simulink model "SO3_model_AIS"  (R2022a)
settings: Solver=ode4  StartTime=0.0  StopTime=180  FixedStep=0.02  RelTol=1e-3
values from neighbouring files (symbols this model uses):
  alpha = 0.05    [Ini_SO3.m]    (also in Ini_SO3_MixedCZ.m = 0.3; coneNew.m = acos(cosalpha))
  alpha1 = 0.25    [Ini_SO3.m]
  beta = 0.05    [Ini_SO3.m]    (also in Ini_SO3_MixedCZ.m = 0.3)
  deltar = 0.005    [Ini_SO3.m]    (also in Ini_SO3_MixedCZ.m = 0.01; Ini_Usat.m = 0.01)
  G = [1,0,0 ... (first row only)    [Ini_SO3.m]    (also in Ini_SO3_MixedCZ.m; Symmetric test.m = inv(J)*D*E*D')
  J0 = [60 0 -5 ... (first row only)    [Ini_SO3.m]    (also in Ini_SO3_MixedCZ.m)
  J1 = [60 0 -5 ... (first row only)    [Ini_SO3.m]    (also in Ini_SO3_MixedCZ.m)
  J2 = [60 0 -5 ... (first row only)    [Ini_SO3.m]    (also in Ini_SO3_MixedCZ.m)
  J3 = [60 0 -5 ... (first row only)    [Ini_SO3.m]    (also in Ini_SO3_MixedCZ.m)
  K1 = [0.01,0,30,0.2]'    [Ini_SO3.m]    (also in Ini_SO3_MixedCZ.m = [0.01,0,30,0.1]')
  K2 = [0.01,55,55,16,0.001,0.001,0.001]'    [Ini_SO3.m]
  lambda = 0.05    [Ini_SO3.m]    (also in Ini_SO3_MixedCZ.m = 0.3; SO3toThetan.m = diag(lambda))
  lambda1 = 0.25    [Ini_SO3.m]
  N = R/deltar    (= 200)    [Ini_SO3.m]    (also in Ini_SO3_MixedCZ.m; Ini_Usat.m)
  Omega01 = [0.03;0.02;-0.03]    [Ini_SO3.m]    (also in Ini_SO3_MixedCZ.m = [0,0,0])
  Omega02 = [-0.02;0.02;-0.03]    [Ini_SO3.m]    (also in Ini_SO3_MixedCZ.m = [0,0,0])
  Omega03 = [0;0.03;0.04]    [Ini_SO3.m]    (also in Ini_SO3_MixedCZ.m = [0,0,0])
  Omega0d = [0;0;0]    [Ini_SO3.m]    (also in Ini_SO3_MixedCZ.m)
  R = 1    [Ini_SO3.m]    (also in Ini_SO3_MixedCZ.m = 2; Ini_Usat.m = 2; SO3.m = eye(3)+(1-cos(ang))*x2x_hat(x)*x2x_hat(x)+sin(ang)*x2x_hat(x; plot2D.m = tran(lamda_con(j),phi_con(j)))
  R01 = SO3(deg2rad(-80), nd0)    [Ini_SO3.m]    (also in Ini_SO3_MixedCZ.m = SO3(2.387, [0.3145,0.9113,0.2658]'))
  R02 = SO3(deg2rad(40),[0;1;1]/norm([0;1;1]))    [Ini_SO3.m]    (also in Ini_SO3_MixedCZ.m = SO3(1.422, [0.1772,0.9751,-0.1329]'))
  R03 = SO3(deg2rad(-120), nd0)    [Ini_SO3.m]    (also in Ini_SO3_MixedCZ.m = SO3(2.007, [0.2997,0.9415,0.1543]'))
  Rd = SO3(-(2*pi-Angd),nd)    [Ini_SO3.m]    (also in Ini_SO3_MixedCZ.m = SO3(Angd,nd))
  Rd0 = SO3(-(2*pi-Angd0),nd0)    [Ini_SO3.m]    (also in Ini_SO3_MixedCZ.m = SO3(Angd0,nd0))
  thate_T = deg2rad(30)    [Ini_SO3.m]    (also in Ini_SO3_MixedCZ.m = deg2rad(10))
  X = zeros(4,4)    [Ini_SO3.m]    (also in Ini_SO3_MixedCZ.m; coneNew.m = R .* cos(A))
undefined symbols (not defined in the file or in its folder): deg, rad, s
libraries: matrix_library x7, aerolibconvert2 x5
(part 1 of 2)
settings Model: Creator=Zeyu  LastModifiedBy=泽禹
settings DebuggingCC: UnconnectedInputMsg=warning  UnconnectedOutputMsg=warning  UnconnectedLineMsg=warning  UnderSpecifiedDimensionMsg=warning
settings RTWCC: DLArmComputeVersion=19.05

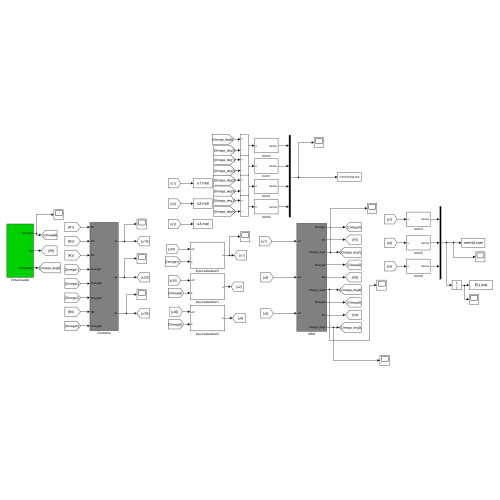
[thumbnail: Simulink's stored preview of the top-level diagram]
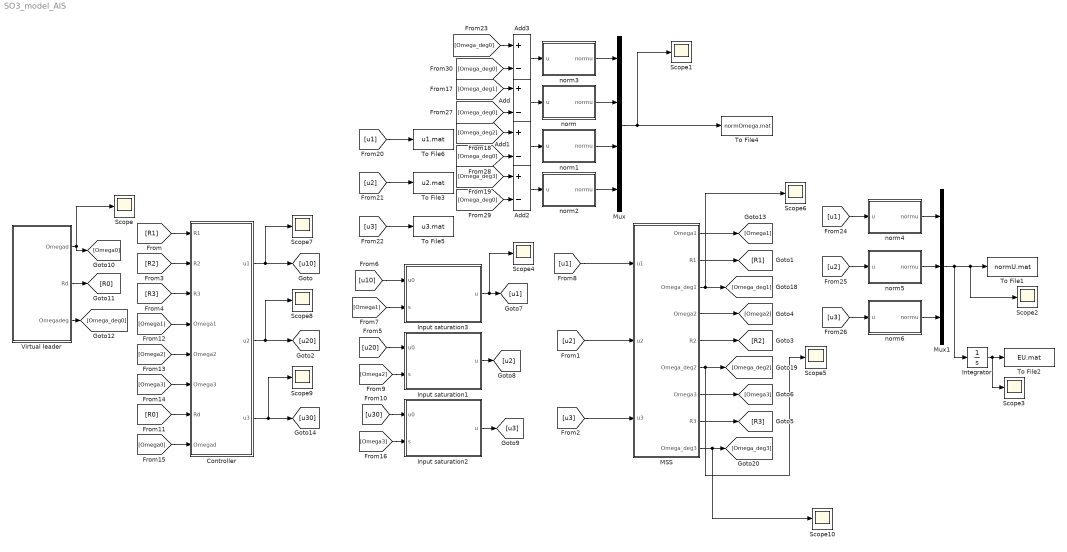
== system SO3_model_AIS ==
  Add{,1..3} (4 alike) : Sum  Inputs=+-
  Controller : Subsystem
  Input saturation1 : Subsystem
  Input saturation2 : Subsystem
  Input saturation3 : Subsystem
  Integrator : Integrator
  MSS : Subsystem
  Mux : Mux
  Mux1 : Mux  Inputs=3
  Scope{,1..10} (11 alike) : Scope
  To File1 : ToFile  Filename=normU.mat  MatrixName=normU
  To File2 : ToFile  Filename=EU.mat  MatrixName=EU
  To File3 : ToFile  Filename=u2.mat  MatrixName=u2
  To File4 : ToFile  Filename=normOmega.mat  MatrixName=normOmega
  To File5 : ToFile  Filename=u3.mat  MatrixName=u3
  To File6 : ToFile  Filename=u1.mat  MatrixName=u1
  Virtual leader : Subsystem
  norm : Subsystem
  norm1 : Subsystem
  norm2 : Subsystem
  norm3 : Subsystem
  norm4 : Subsystem
  norm5 : Subsystem
  norm6 : Subsystem
  wires:
  Virtual leader/1(Omegad) -> [Omega0], Scope/1
  Virtual leader/2(Rd) -> [R0]
  [R1] -> Controller/1(R1)
  [R2] -> Controller/2(R2)
  [R3] -> Controller/3(R3)
  [Omega1] -> Controller/4(Omega1)
  [Omega2] -> Controller/5(Omega2)
  [Omega3] -> Controller/6(Omega3)
  [R0] -> Controller/7(Rd)
  [Omega0] -> Controller/8(Omegad)
  Controller/1(u1) -> Scope7/1, [u10]
  Controller/2(u2) -> Scope8/1, [u20]
  Controller/3(u3) -> Scope9/1, [u30]
  MSS/1(Omega1) -> [Omega1]
  MSS/2(R1) -> [R1]
  MSS/3(Omega_deg1) -> Scope6/1, [Omega_deg1]
  MSS/4(Omega2) -> [Omega2]
  MSS/5(R2) -> [R2]
  MSS/7(Omega3) -> [Omega3]
  MSS/8(R3) -> [R3]
  MSS/9(Omega_deg3) -> Scope10/1, [Omega_deg3]
  [u10] -> Input saturation3/1(u0)
  [Omega1] -> Input saturation3/2(s)
  Input saturation3/1(u) -> Scope4/1, [u1]
  [u20] -> Input saturation1/1(u0)
  [Omega2] -> Input saturation1/2(s)
  Input saturation1/1(u) -> [u2]
  [u30] -> Input saturation2/1(u0)
  [Omega3] -> Input saturation2/2(s)
  Input saturation2/1(u) -> [u3]
  [u1] -> MSS/1(u1)
  [u2] -> MSS/2(u2)
  [u3] -> MSS/3(u3)
  MSS/6(Omega_deg2) -> Scope5/1, [Omega_deg2]
  [u1] -> To File6/1
  [u3] -> To File5/1
  [u2] -> To File3/1
  Virtual leader/3(Omegadeg) -> [Omega_deg0]
  norm3/1(normu) -> Mux/1
  norm/1(normu) -> Mux/2
  norm1/1(normu) -> Mux/3
  norm2/1(normu) -> Mux/4
  Mux/1 -> Scope1/1, To File4/1
  norm4/1(normu) -> Mux1/1
  norm5/1(normu) -> Mux1/2
  norm6/1(normu) -> Mux1/3
  [u1] -> norm4/1(u)
  [u2] -> norm5/1(u)
  [u3] -> norm6/1(u)
  Mux1/1 -> Integrator/1, Scope2/1, To File1/1
  Integrator/1 -> Scope3/1, To File2/1
  [Omega_deg1] -> Add/1
  Add/1 -> norm/1(u)
  [Omega_deg0] -> Add/2
  [Omega_deg0] -> Add1/2
  [Omega_deg2] -> Add1/1
  Add1/1 -> norm1/1(u)
  [Omega_deg0] -> Add2/2
  [Omega_deg3] -> Add2/1
  Add2/1 -> norm2/1(u)
  [Omega_deg0] -> Add3/2
  Add3/1 -> norm3/1(u)
  [Omega_deg0] -> Add3/1

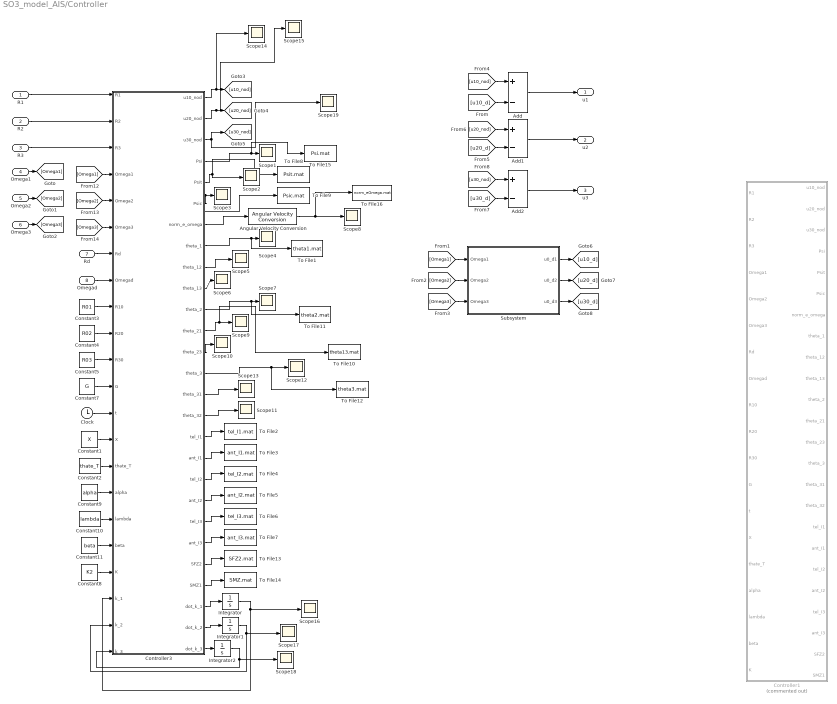
== system SO3_model_AIS/Controller ==
  R1 : Inport
  R2 : Inport  Port=2
  R3 : Inport  Port=3
  Omega1 : Inport  Port=4
  Omega2 : Inport  Port=5
  Omega3 : Inport  Port=6
  Rd : Inport  Port=7
  Omegad : Inport  Port=8
  Add : Sum  Inputs=+-
  Add1 : Sum  Inputs=+-
  Add2 : Sum  Inputs=+-
  Angular Velocity Conversion : aerolibconvert2/Angular Velocity Conversion  IU=rad/s  OU=deg/s
  Clock : Clock
  Constant1 : Constant  Value=X
  Constant10 : Constant  Value=lambda
  Constant11 : Constant  Value=beta
  Constant2 : Constant  Value=thate_T
  Constant3 : Constant  Value=R01
  Constant4 : Constant  Value=R02
  Constant5 : Constant  Value=R03
  Constant7 : Constant  Value=G
  Constant8 : Constant  Value=K2
  Constant9 : Constant  Value=alpha
  Controller1 : MATLAB Function  Commented=on  TreatAsAtomicUnit=on
  Controller3 : MATLAB Function  TreatAsAtomicUnit=on
  Integrator : Integrator  InitialCondition=[0.05;0.05;0.05]
  Integrator1 : Integrator  InitialCondition=[0.05;0.05;0.05]
  Integrator2 : Integrator  InitialCondition=[0.05;0.05;0.05]
  Scope{1..19} (19 alike) : Scope
  Subsystem : Subsystem
  To File1 : ToFile  Filename=theta1.mat  MatrixName=theta1
  To File10 : ToFile  Filename=theta13.mat  MatrixName=theta13
  To File11 : ToFile  Filename=theta2.mat  MatrixName=theta2
  To File12 : ToFile  Filename=theta3.mat  MatrixName=theta3
  To File13 : ToFile  Filename=SFZ2.mat  MatrixName=SFZ2
  To File14 : ToFile  Filename=SMZ.mat  MatrixName=SMZ
  To File15 : ToFile  Filename=Psi.mat  MatrixName=Psi
  To File16 : ToFile  Filename=norm_eOmega.mat  MatrixName=norm_eOmega
  To File2 : ToFile  Filename=tel_I1.mat  MatrixName=tel_I1
  To File3 : ToFile  Filename=ant_I1.mat  MatrixName=ant_I1
  To File4 : ToFile  Filename=tel_I2.mat  MatrixName=tel_I2
  To File5 : ToFile  Filename=ant_I2.mat  MatrixName=ant_I2
  To File6 : ToFile  Filename=tel_I3.mat  MatrixName=tel_I3
  To File7 : ToFile  Filename=ant_I3.mat  MatrixName=ant_I3
  To File8 : ToFile  Filename=Psit.mat  MatrixName=Psit
  To File9 : ToFile  Filename=Psic.mat  MatrixName=Psic
  u1 : Outport
  u2 : Outport  Port=2
  u3 : Outport  Port=3
  wires:
  Constant7/1 -> Controller3/12(G)
  Clock/1 -> Controller3/13(t)
  Constant8/1 -> Controller3/19(K)
  Constant4/1 -> Controller3/10(R20)
  Constant10/1 -> Controller3/17(lambda)
  Constant3/1 -> Controller3/9(R10)
  Omegad/1 -> Controller3/8(Omegad)
  R2/1 -> Controller3/2(R2)
  Constant11/1 -> Controller3/18(beta)
  Constant2/1 -> Controller3/15(thate_T)
  Constant1/1 -> Controller3/14(X)
  Controller3/7(norm_e_omega) -> Angular Velocity Conversion/1
  Constant9/1 -> Controller3/16(alpha)
  Rd/1 -> Controller3/7(Rd)
  Controller3/4(Psi) -> Scope1/1, To File15/1
  Controller3/6(Psic) -> To File9/1, Scope3/1
  R3/1 -> Controller3/3(R3)
  Constant5/1 -> Controller3/11(R30)
  R1/1 -> Controller3/1(R1)
  [Omega2] -> Controller3/5(Omega2)
  [Omega1] -> Controller3/4(Omega1)
  [Omega3] -> Controller3/6(Omega3)
  Omega1/1 -> [Omega1]
  Omega2/1 -> [Omega2]
  Omega3/1 -> [Omega3]
  [Omega1] -> Subsystem/1(Omega1)
  [Omega2] -> Subsystem/2(Omega2)
  [Omega3] -> Subsystem/3(Omega3)
  Add/1 -> u1/1
  Add1/1 -> u2/1
  Add2/1 -> u3/1
  Controller3/1(u10_nod) -> Scope14/1, [u10_nod]
  Controller3/2(u20_nod) -> Scope15/1, [u20_nod]
  Controller3/3(u30_nod) -> [u30_nod], Scope19/1
  Subsystem/2(u0_d2) -> [u20_d]
  Subsystem/1(u0_d1) -> [u10_d]
  Subsystem/3(u0_d3) -> [u30_d]
  [u10_d] -> Add/2
  [u10_nod] -> Add/1
  [u20_d] -> Add1/2
  [u20_nod] -> Add1/1
  [u30_d] -> Add2/2
  [u30_nod] -> Add2/1
  Controller3/17(tel_I1) -> To File2/1
  Controller3/18(ant_I1) -> To File3/1
  Controller3/19(tel_I2) -> To File4/1
  Controller3/20(ant_I2) -> To File5/1
  Controller3/21(tel_I3) -> To File6/1
  Controller3/22(ant_I3) -> To File7/1
  Controller3/8(theta_1) -> To File1/1, Scope4/1
  Controller3/9(theta_12) -> Scope5/1
  Controller3/12(theta_21) -> To File10/1, Scope9/1
  Controller3/13(theta_23) -> Scope10/1
  Controller3/16(theta_32) -> Scope11/1
  Controller3/15(theta_31) -> Scope13/1
  Controller3/14(theta_3) -> To File12/1, Scope12/1
  Controller3/5(Psit) -> Scope2/1, To File8/1
  Controller3/10(theta_13) -> Scope6/1
  Controller3/11(theta_2) -> To File11/1, Scope7/1
  Controller3/23(SFZ2) -> To File13/1
  Controller3/24(SMZ1) -> To File14/1
  Controller3/25(dot_k_1) -> Integrator/1
  Integrator/1 -> Scope16/1, Controller3/20(k_1)
  Controller3/26(dot_k_2) -> Integrator1/1
  Integrator1/1 -> Scope17/1, Controller3/21(k_2)
  Controller3/27(dot_k_3) -> Integrator2/1
  Integrator2/1 -> Scope18/1, Controller3/22(k_3)
  Angular Velocity Conversion/1 -> To File16/1, Scope8/1

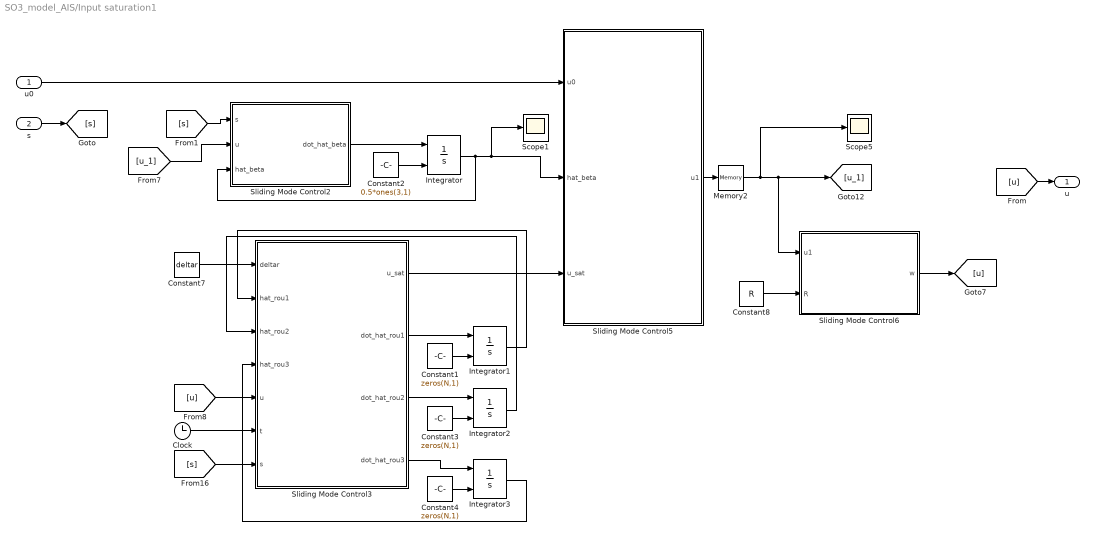
== system SO3_model_AIS/Input saturation1 ==
  u0 : Inport
  s : Inport  Port=2
  Clock : Clock
  Constant1 : Constant  Value=zeros(N,1)
  Constant2 : Constant  Value=0.5*ones(3,1)
  Constant3 : Constant  Value=zeros(N,1)
  Constant4 : Constant  Value=zeros(N,1)
  Constant7 : Constant  Value=deltar
  Constant8 : Constant  Value=R
  Integrator{,1..3} (4 alike) : Integrator  InitialConditionSource=external
  Memory2 : Memory
  Scope1 : Scope
  Scope5 : Scope
  Sliding Mode Control2 : MATLAB Function  TreatAsAtomicUnit=on
  Sliding Mode Control3 : MATLAB Function  TreatAsAtomicUnit=on
  Sliding Mode Control5 : MATLAB Function  TreatAsAtomicUnit=on
  Sliding Mode Control6 : MATLAB Function  TreatAsAtomicUnit=on
  u : Outport
  wires:
  [s] -> Sliding Mode Control2/1(s)
  s/1 -> [s]
  [u] -> u/1
  u0/1 -> Sliding Mode Control5/1(u0)
  Constant8/1 -> Sliding Mode Control6/2(R)
  Memory2/1 -> Scope5/1, Sliding Mode Control6/1(u1), [u_1]
  Sliding Mode Control6/1(w) -> [u]
  [u_1] -> Sliding Mode Control2/2(u)
  Sliding Mode Control5/1(u1) -> Memory2/1
  Sliding Mode Control2/1(dot_hat_beta) -> Integrator/1
  Constant2/1 -> Integrator/2
  Integrator/1 -> Sliding Mode Control2/3(hat_beta), Scope1/1, Sliding Mode Control5/2(hat_beta)
  [u] -> Sliding Mode Control3/5(u)
  Integrator1/1 -> Sliding Mode Control3/2(hat_rou1)
  Sliding Mode Control3/3(dot_hat_rou2) -> Integrator2/1
  [s] -> Sliding Mode Control3/7(s)
  Constant7/1 -> Sliding Mode Control3/1(deltar)
  Constant4/1 -> Integrator3/2
  Integrator2/1 -> Sliding Mode Control3/3(hat_rou2)
  Sliding Mode Control3/4(dot_hat_rou3) -> Integrator3/1
  Integrator3/1 -> Sliding Mode Control3/4(hat_rou3)
  Sliding Mode Control3/2(dot_hat_rou1) -> Integrator1/1
  Clock/1 -> Sliding Mode Control3/6(t)
  Constant1/1 -> Integrator1/2
  Sliding Mode Control3/1(u_sat) -> Sliding Mode Control5/3(u_sat)
  Constant3/1 -> Integrator2/2

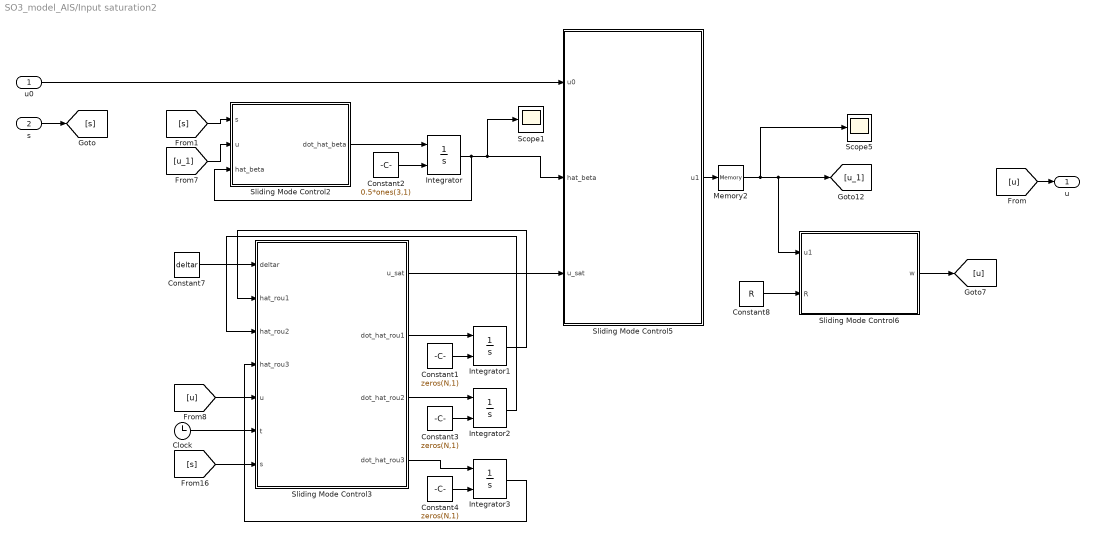
== system SO3_model_AIS/Input saturation2 ==
  u0 : Inport
  s : Inport  Port=2
  Clock : Clock
  Constant1 : Constant  Value=zeros(N,1)
  Constant2 : Constant  Value=0.5*ones(3,1)
  Constant3 : Constant  Value=zeros(N,1)
  Constant4 : Constant  Value=zeros(N,1)
  Constant7 : Constant  Value=deltar
  Constant8 : Constant  Value=R
  Integrator{,1..3} (4 alike) : Integrator  InitialConditionSource=external
  Memory2 : Memory
  Scope1 : Scope
  Scope5 : Scope
  Sliding Mode Control2 : MATLAB Function  TreatAsAtomicUnit=on
  Sliding Mode Control3 : MATLAB Function  TreatAsAtomicUnit=on
  Sliding Mode Control5 : MATLAB Function  TreatAsAtomicUnit=on
  Sliding Mode Control6 : MATLAB Function  TreatAsAtomicUnit=on
  u : Outport
  wires:
  Constant2/1 -> Integrator/2
  Sliding Mode Control2/1(dot_hat_beta) -> Integrator/1
  Sliding Mode Control5/1(u1) -> Memory2/1
  [u_1] -> Sliding Mode Control2/2(u)
  Sliding Mode Control6/1(w) -> [u]
  Memory2/1 -> Sliding Mode Control6/1(u1), [u_1], Scope5/1
  Constant8/1 -> Sliding Mode Control6/2(R)
  [u] -> u/1
  s/1 -> [s]
  [s] -> Sliding Mode Control2/1(s)
  Integrator/1 -> Sliding Mode Control2/3(hat_beta), Scope1/1, Sliding Mode Control5/2(hat_beta)
  u0/1 -> Sliding Mode Control5/1(u0)
  [u] -> Sliding Mode Control3/5(u)
  Integrator1/1 -> Sliding Mode Control3/2(hat_rou1)
  Sliding Mode Control3/3(dot_hat_rou2) -> Integrator2/1
  [s] -> Sliding Mode Control3/7(s)
  Constant7/1 -> Sliding Mode Control3/1(deltar)
  Constant4/1 -> Integrator3/2
  Integrator2/1 -> Sliding Mode Control3/3(hat_rou2)
  Sliding Mode Control3/4(dot_hat_rou3) -> Integrator3/1
  Sliding Mode Control3/2(dot_hat_rou1) -> Integrator1/1
  Clock/1 -> Sliding Mode Control3/6(t)
  Constant1/1 -> Integrator1/2
  Sliding Mode Control3/1(u_sat) -> Sliding Mode Control5/3(u_sat)
  Constant3/1 -> Integrator2/2
  Integrator3/1 -> Sliding Mode Control3/4(hat_rou3)

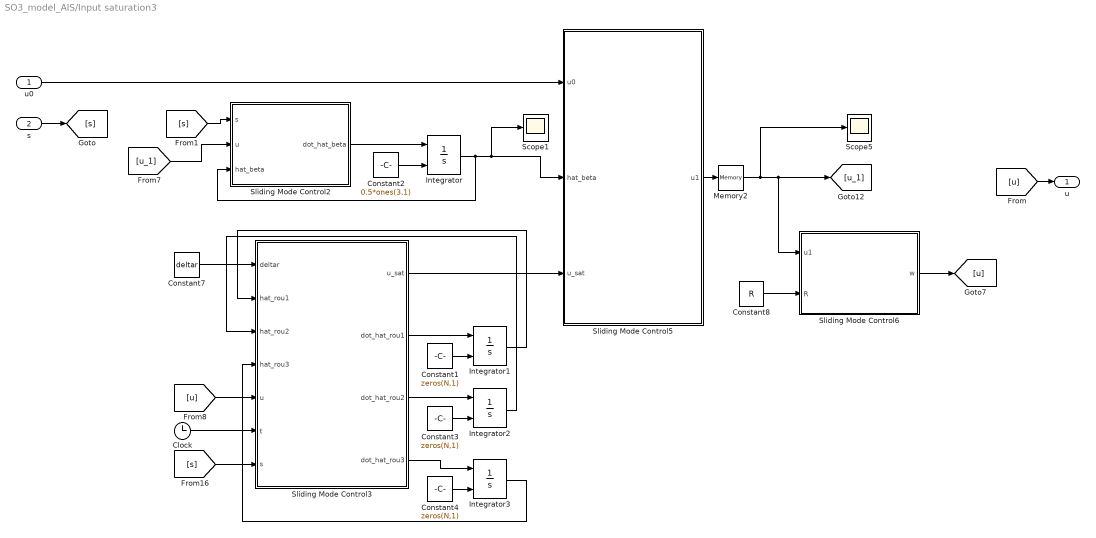
== system SO3_model_AIS/Input saturation3 ==
  u0 : Inport
  s : Inport  Port=2
  Clock : Clock
  Constant1 : Constant  Value=zeros(N,1)
  Constant2 : Constant  Value=0.5*ones(3,1)
  Constant3 : Constant  Value=zeros(N,1)
  Constant4 : Constant  Value=zeros(N,1)
  Constant7 : Constant  Value=deltar
  Constant8 : Constant  Value=R
  Integrator{,1..3} (4 alike) : Integrator  InitialConditionSource=external
  Memory2 : Memory
  Scope1 : Scope
  Scope5 : Scope
  Sliding Mode Control2 : MATLAB Function  TreatAsAtomicUnit=on
  Sliding Mode Control3 : MATLAB Function  TreatAsAtomicUnit=on
  Sliding Mode Control5 : MATLAB Function  TreatAsAtomicUnit=on
  Sliding Mode Control6 : MATLAB Function  TreatAsAtomicUnit=on
  u : Outport
  wires:
  Constant3/1 -> Integrator2/2
  Sliding Mode Control3/1(u_sat) -> Sliding Mode Control5/3(u_sat)
  Constant1/1 -> Integrator1/2
  Clock/1 -> Sliding Mode Control3/6(t)
  Sliding Mode Control3/2(dot_hat_rou1) -> Integrator1/1
  Integrator3/1 -> Sliding Mode Control3/4(hat_rou3)
  Sliding Mode Control3/4(dot_hat_rou3) -> Integrator3/1
  Integrator2/1 -> Sliding Mode Control3/3(hat_rou2)
  Constant4/1 -> Integrator3/2
  Constant7/1 -> Sliding Mode Control3/1(deltar)
  [s] -> Sliding Mode Control3/7(s)
  Sliding Mode Control3/3(dot_hat_rou2) -> Integrator2/1
  Integrator1/1 -> Sliding Mode Control3/2(hat_rou1)
  [u] -> Sliding Mode Control3/5(u)
  Integrator/1 -> Sliding Mode Control5/2(hat_beta), Scope1/1, Sliding Mode Control2/3(hat_beta)
  Constant2/1 -> Integrator/2
  Sliding Mode Control2/1(dot_hat_beta) -> Integrator/1
  Sliding Mode Control5/1(u1) -> Memory2/1
  [u_1] -> Sliding Mode Control2/2(u)
  Sliding Mode Control6/1(w) -> [u]
  Memory2/1 -> [u_1], Sliding Mode Control6/1(u1), Scope5/1
  Constant8/1 -> Sliding Mode Control6/2(R)
  u0/1 -> Sliding Mode Control5/1(u0)
  [u] -> u/1
  s/1 -> [s]
  [s] -> Sliding Mode Control2/1(s)

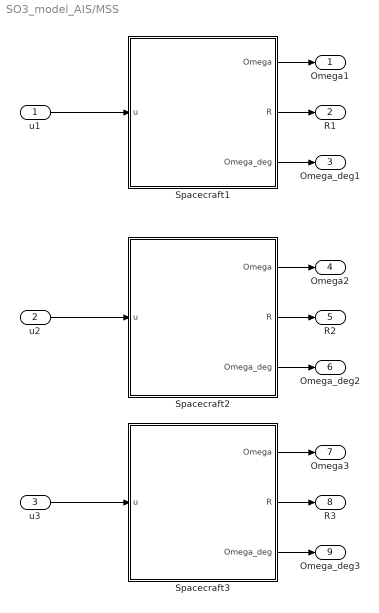
== system SO3_model_AIS/MSS ==
  u1 : Inport
  u2 : Inport  Port=2
  u3 : Inport  Port=3
  Spacecraft1 : Subsystem
  Spacecraft2 : Subsystem
  Spacecraft3 : Subsystem
  Omega1 : Outport
  R1 : Outport  Port=2
  Omega_deg1 : Outport  Port=3
  Omega2 : Outport  Port=4
  R2 : Outport  Port=5
  Omega_deg2 : Outport  Port=6
  Omega3 : Outport  Port=7
  R3 : Outport  Port=8
  Omega_deg3 : Outport  Port=9
  wires:
  Spacecraft3/2(R) -> R3/1
  Spacecraft1/1(Omega) -> Omega1/1
  u1/1 -> Spacecraft1/1(u)
  Spacecraft2/3(Omega_deg) -> Omega_deg2/1
  Spacecraft2/1(Omega) -> Omega2/1
  u3/1 -> Spacecraft3/1(u)
  Spacecraft1/2(R) -> R1/1
  Spacecraft3/3(Omega_deg) -> Omega_deg3/1
  Spacecraft3/1(Omega) -> Omega3/1
  Spacecraft1/3(Omega_deg) -> Omega_deg1/1
  u2/1 -> Spacecraft2/1(u)
  Spacecraft2/2(R) -> R2/1

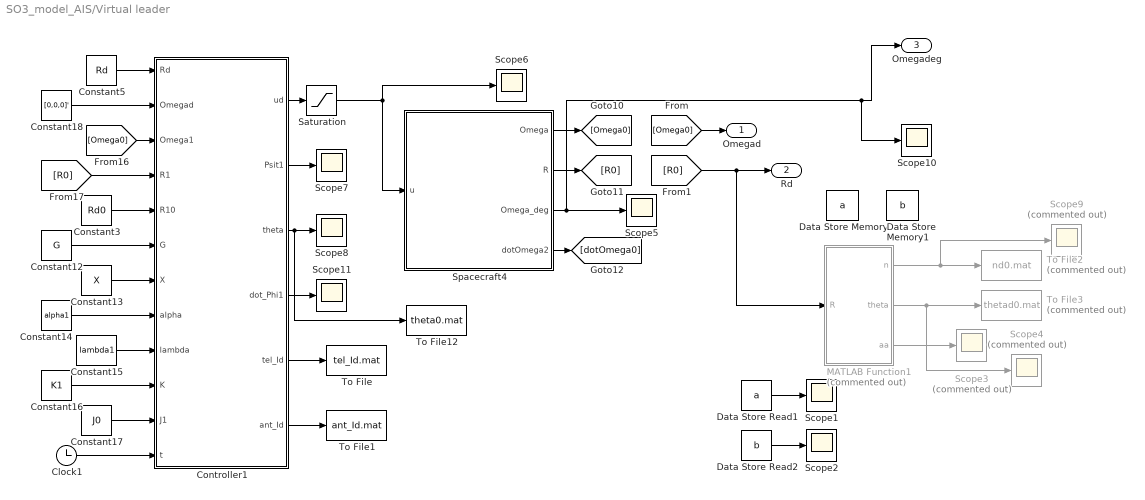
== system SO3_model_AIS/Virtual leader ==
  Clock1 : Clock
  Constant12 : Constant  Value=G
  Constant13 : Constant  Value=X
  Constant14 : Constant  Value=alpha1
  Constant15 : Constant  Value=lambda1
  Constant16 : Constant  Value=K1
  Constant17 : Constant  Value=J0
  Constant18 : Constant  Value=[0,0,0]'
  Constant3 : Constant  Value=Rd0
  Constant5 : Constant  Value=Rd
  Controller1 : MATLAB Function  TreatAsAtomicUnit=on
  Data Store Memory : DataStoreMemory  DataStoreName=a  ReadBeforeWriteMsg=warning  WriteAfterWriteMsg=warning  WriteAfterReadMsg=warning  InitialValue=ones(4,1)  ShowAdditionalParam=off  OutDataTypeStr=double
  Data Store Memory1 : DataStoreMemory  DataStoreName=b  ReadBeforeWriteMsg=warning  WriteAfterWriteMsg=warning  WriteAfterReadMsg=warning  InitialValue=zeros(4,1)  ShowAdditionalParam=off  OutDataTypeStr=double
  Data Store Read1 : DataStoreRead  DataStoreName=a  IndexOptions=Index vector (dialog)  Indices=1  OutputSizes=1
  Data Store Read2 : DataStoreRead  DataStoreName=b  IndexOptions=Index vector (dialog)  Indices=1  OutputSizes=1
  MATLAB Function1 : MATLAB Function  Commented=on  TreatAsAtomicUnit=on
  Saturation : Saturate  UpperLimit=1  LowerLimit=-1
  Scope{1..2,5..8,10..11} (8 alike) : Scope
  Scope3 : Scope  Commented=on
  Scope4 : Scope  Commented=on
  Scope9 : Scope  Commented=on
  Spacecraft4 : Subsystem
  To File : ToFile  Filename=tel_Id.mat  MatrixName=tel_Id
  To File1 : ToFile  Filename=ant_Id.mat  MatrixName=ant_Id
  To File12 : ToFile  Filename=theta0.mat  MatrixName=theta0
  To File2 : ToFile  Commented=on  Filename=nd0.mat  MatrixName=nd0
  To File3 : ToFile  Commented=on  Filename=thetad0.mat  MatrixName=thetad0
  Omegad : Outport
  Rd : Outport  Port=2
  Omegadeg : Outport  Port=3
  wires:
  Spacecraft4/4(dotOmega2) -> [dotOmega0]
  [R0] -> Controller1/4(R1)
  Controller1/1(ud) -> Saturation/1
  Constant16/1 -> Controller1/10(K)
  Constant12/1 -> Controller1/6(G)
  Constant18/1 -> Controller1/2(Omegad)
  Constant17/1 -> Controller1/11(J1)
  Constant5/1 -> Controller1/1(Rd)
  Constant14/1 -> Controller1/8(alpha)
  Constant15/1 -> Controller1/9(lambda)
  Constant13/1 -> Controller1/7(X)
  Clock1/1 -> Controller1/12(t)
  [Omega0] -> Controller1/3(Omega1)
  Controller1/4(dot_Phi1) -> Scope11/1
  Controller1/2(Psit1) -> Scope7/1
  Spacecraft4/2(R) -> [R0]
  Spacecraft4/1(Omega) -> [Omega0]
  [Omega0] -> Omegad/1
  Constant3/1 -> Controller1/5(R10)
  Data Store Read1/1 -> Scope1/1
  Data Store Read2/1 -> Scope2/1
  Saturation/1 -> Spacecraft4/1(u), Scope6/1
  Controller1/5(tel_Id) -> To File/1
  Controller1/6(ant_Id) -> To File1/1
  [R0] -> MATLAB Function1/1(R), Rd/1
  MATLAB Function1/1(n) -> Scope9/1, To File2/1
  MATLAB Function1/2(theta) -> Scope4/1, To File3/1
  MATLAB Function1/3(aa) -> Scope3/1
  Controller1/3(theta) -> To File12/1, Scope8/1
  Spacecraft4/3(Omega_deg) -> Scope5/1, Scope10/1, Omegadeg/1

== system SO3_model_AIS/norm ==
  u : Inport
  Matrix Square : matrix_library/Matrix Square  OutMin=[]  OutMax=[]
      settings: SourceProductBaseCode=DS
  Sqrt : Sqrt
  normu : Outport
  wires:
  Sqrt/1 -> normu/1
  Matrix Square/1 -> Sqrt/1
  u/1 -> Matrix Square/1

== system SO3_model_AIS/norm1 ==
  u : Inport
  Matrix Square : matrix_library/Matrix Square  OutMin=[]  OutMax=[]
      settings: SourceProductBaseCode=DS
  Sqrt : Sqrt
  normu : Outport
  wires:
  Sqrt/1 -> normu/1
  Matrix Square/1 -> Sqrt/1
  u/1 -> Matrix Square/1

== system SO3_model_AIS/norm2 ==
  u : Inport
  Matrix Square : matrix_library/Matrix Square  OutMin=[]  OutMax=[]
      settings: SourceProductBaseCode=DS
  Sqrt : Sqrt
  normu : Outport
  wires:
  Sqrt/1 -> normu/1
  Matrix Square/1 -> Sqrt/1
  u/1 -> Matrix Square/1

== system SO3_model_AIS/norm3 ==
  u : Inport
  Matrix Square : matrix_library/Matrix Square  OutMin=[]  OutMax=[]
      settings: SourceProductBaseCode=DS
  Sqrt : Sqrt
  normu : Outport
  wires:
  u/1 -> Matrix Square/1
  Matrix Square/1 -> Sqrt/1
  Sqrt/1 -> normu/1

== system SO3_model_AIS/norm4 ==
  u : Inport
  Matrix Square : matrix_library/Matrix Square  OutMin=[]  OutMax=[]
      settings: SourceProductBaseCode=DS
  Sqrt : Sqrt
  normu : Outport
  wires:
  Sqrt/1 -> normu/1
  Matrix Square/1 -> Sqrt/1
  u/1 -> Matrix Square/1

== system SO3_model_AIS/norm5 ==
  u : Inport
  Matrix Square : matrix_library/Matrix Square  OutMin=[]  OutMax=[]
      settings: SourceProductBaseCode=DS
  Sqrt : Sqrt
  normu : Outport
  wires:
  u/1 -> Matrix Square/1
  Matrix Square/1 -> Sqrt/1
  Sqrt/1 -> normu/1

== system SO3_model_AIS/norm6 ==
  u : Inport
  Matrix Square : matrix_library/Matrix Square  OutMin=[]  OutMax=[]
      settings: SourceProductBaseCode=DS
  Sqrt : Sqrt
  normu : Outport
  wires:
  Sqrt/1 -> normu/1
  Matrix Square/1 -> Sqrt/1
  u/1 -> Matrix Square/1

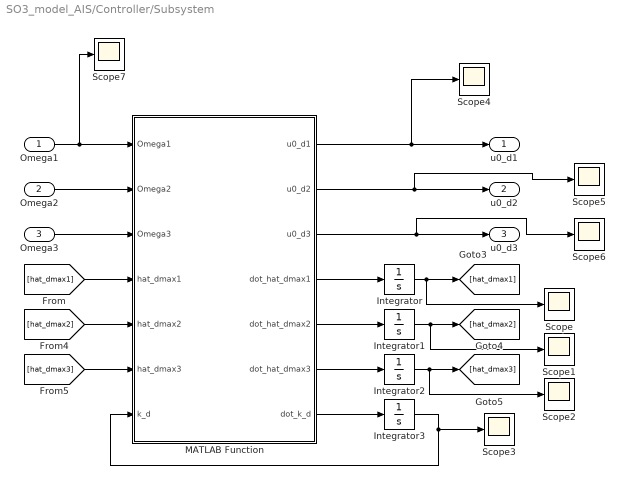
== system SO3_model_AIS/Controller/Subsystem ==
  Omega1 : Inport
  Omega2 : Inport  Port=2
  Omega3 : Inport  Port=3
  Integrator : Integrator
  Integrator1 : Integrator
  Integrator2 : Integrator
  Integrator3 : Integrator  InitialCondition=0.05*ones(3,1)
  MATLAB Function : MATLAB Function  TreatAsAtomicUnit=on
  Scope{,1..7} (8 alike) : Scope
  u0_d1 : Outport
  u0_d2 : Outport  Port=2
  u0_d3 : Outport  Port=3
  wires:
  Integrator2/1 -> [hat_dmax3], Scope2/1
  Integrator1/1 -> Scope1/1, [hat_dmax2]
  MATLAB Function/1(u0_d1) -> Scope4/1, u0_d1/1
  MATLAB Function/4(dot_hat_dmax1) -> Integrator/1
  [hat_dmax2] -> MATLAB Function/5(hat_dmax2)
  MATLAB Function/5(dot_hat_dmax2) -> Integrator1/1
  Omega2/1 -> MATLAB Function/2(Omega2)
  Omega1/1 -> Scope7/1, MATLAB Function/1(Omega1)
  [hat_dmax3] -> MATLAB Function/6(hat_dmax3)
  MATLAB Function/6(dot_hat_dmax3) -> Integrator2/1
  Integrator/1 -> Scope/1, [hat_dmax1]
  [hat_dmax1] -> MATLAB Function/4(hat_dmax1)
  MATLAB Function/2(u0_d2) -> Scope5/1, u0_d2/1
  MATLAB Function/3(u0_d3) -> Scope6/1, u0_d3/1
  Omega3/1 -> MATLAB Function/3(Omega3)
  MATLAB Function/7(dot_k_d) -> Integrator3/1
  Integrator3/1 -> MATLAB Function/7(k_d), Scope3/1

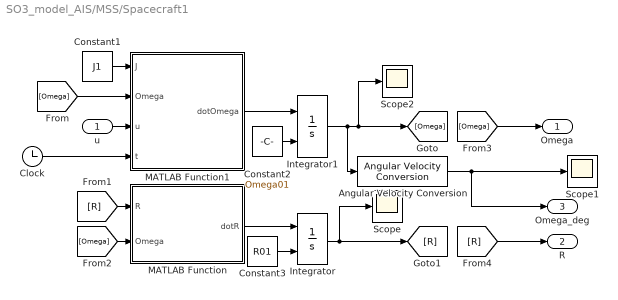
== system SO3_model_AIS/MSS/Spacecraft1 ==
  u : Inport
  Angular Velocity Conversion : aerolibconvert2/Angular Velocity Conversion  IU=rad/s  OU=deg/s
  Clock : Clock
  Constant1 : Constant  Value=J1
  Constant2 : Constant  Value=Omega01
  Constant3 : Constant  Value=R01
  Integrator : Integrator  InitialConditionSource=external
  Integrator1 : Integrator  InitialConditionSource=external
  MATLAB Function : MATLAB Function  TreatAsAtomicUnit=on
  MATLAB Function1 : MATLAB Function  TreatAsAtomicUnit=on
  Scope : Scope
  Scope1 : Scope
  Scope2 : Scope
  Omega : Outport
  R : Outport  Port=2
  Omega_deg : Outport  Port=3
  wires:
  Constant3/1 -> Integrator/2
  Integrator/1 -> [R], Scope/1
  Constant1/1 -> MATLAB Function1/1(J)
  Integrator1/1 -> Scope2/1, [Omega], Angular Velocity Conversion/1
  MATLAB Function1/1(dotOmega) -> Integrator1/1
  [Omega] -> MATLAB Function/2(Omega)
  MATLAB Function/1(dotR) -> Integrator/1
  Constant2/1 -> Integrator1/2
  [Omega] -> MATLAB Function1/2(Omega)
  [R] -> MATLAB Function/1(R)
  Angular Velocity Conversion/1 -> Omega_deg/1, Scope1/1
  u/1 -> MATLAB Function1/3(u)
  [Omega] -> Omega/1
  [R] -> R/1
  Clock/1 -> MATLAB Function1/4(t)

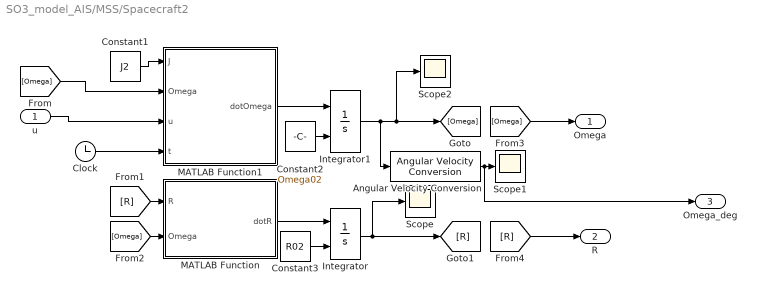
== system SO3_model_AIS/MSS/Spacecraft2 ==
  u : Inport
  Angular Velocity Conversion : aerolibconvert2/Angular Velocity Conversion  IU=rad/s  OU=deg/s
  Clock : Clock
  Constant1 : Constant  Value=J2
  Constant2 : Constant  Value=Omega02
  Constant3 : Constant  Value=R02
  Integrator : Integrator  InitialConditionSource=external
  Integrator1 : Integrator  InitialConditionSource=external
  MATLAB Function : MATLAB Function  TreatAsAtomicUnit=on
  MATLAB Function1 : MATLAB Function  TreatAsAtomicUnit=on
  Scope : Scope
  Scope1 : Scope
  Scope2 : Scope
  Omega : Outport
  R : Outport  Port=2
  Omega_deg : Outport  Port=3
  wires:
  Constant3/1 -> Integrator/2
  Integrator/1 -> [R], Scope/1
  Constant1/1 -> MATLAB Function1/1(J)
  [Omega] -> MATLAB Function/2(Omega)
  MATLAB Function/1(dotR) -> Integrator/1
  Constant2/1 -> Integrator1/2
  [Omega] -> MATLAB Function1/2(Omega)
  [R] -> MATLAB Function/1(R)
  u/1 -> MATLAB Function1/3(u)
  [Omega] -> Omega/1
  [R] -> R/1
  Clock/1 -> MATLAB Function1/4(t)
  Angular Velocity Conversion/1 -> Omega_deg/1, Scope1/1
  Integrator1/1 -> Scope2/1, [Omega], Angular Velocity Conversion/1
  MATLAB Function1/1(dotOmega) -> Integrator1/1

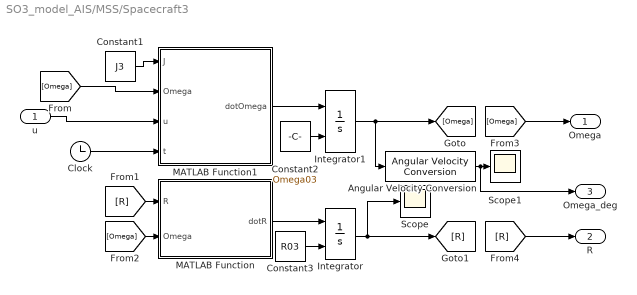
== system SO3_model_AIS/MSS/Spacecraft3 ==
  u : Inport
  Angular Velocity Conversion : aerolibconvert2/Angular Velocity Conversion  IU=rad/s  OU=deg/s
  Clock : Clock
  Constant1 : Constant  Value=J3
  Constant2 : Constant  Value=Omega03
  Constant3 : Constant  Value=R03
  Integrator : Integrator  InitialConditionSource=external
  Integrator1 : Integrator  InitialConditionSource=external
  MATLAB Function : MATLAB Function  TreatAsAtomicUnit=on
  MATLAB Function1 : MATLAB Function  TreatAsAtomicUnit=on
  Scope : Scope
  Scope1 : Scope
  Omega : Outport
  R : Outport  Port=2
  Omega_deg : Outport  Port=3
  wires:
  Constant3/1 -> Integrator/2
  Integrator/1 -> [R], Scope/1
  Constant1/1 -> MATLAB Function1/1(J)
  Integrator1/1 -> [Omega], Angular Velocity Conversion/1
  [Omega] -> MATLAB Function/2(Omega)
  MATLAB Function/1(dotR) -> Integrator/1
  Constant2/1 -> Integrator1/2
  [Omega] -> MATLAB Function1/2(Omega)
  [R] -> MATLAB Function/1(R)
  u/1 -> MATLAB Function1/3(u)
  [Omega] -> Omega/1
  [R] -> R/1
  Clock/1 -> MATLAB Function1/4(t)
  Angular Velocity Conversion/1 -> Omega_deg/1, Scope1/1
  MATLAB Function1/1(dotOmega) -> Integrator1/1

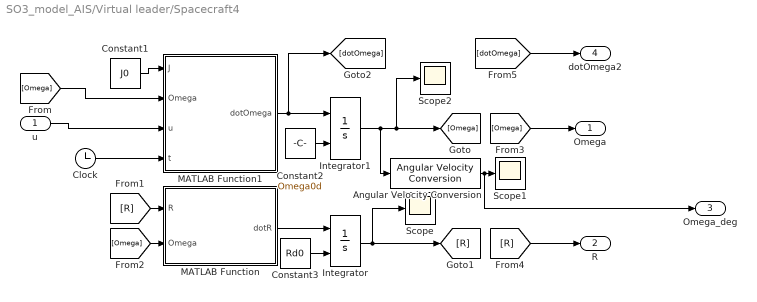
== system SO3_model_AIS/Virtual leader/Spacecraft4 ==
  u : Inport
  Angular Velocity Conversion : aerolibconvert2/Angular Velocity Conversion  IU=rad/s  OU=deg/s
  Clock : Clock
  Constant1 : Constant  Value=J0
  Constant2 : Constant  Value=Omega0d
  Constant3 : Constant  Value=Rd0
  Integrator : Integrator  InitialConditionSource=external
  Integrator1 : Integrator  InitialConditionSource=external
  MATLAB Function : MATLAB Function  TreatAsAtomicUnit=on
  MATLAB Function1 : MATLAB Function  TreatAsAtomicUnit=on
  Scope : Scope
  Scope1 : Scope
  Scope2 : Scope
  Omega : Outport
  R : Outport  Port=2
  Omega_deg : Outport  Port=3
  dotOmega2 : Outport  Port=4
  wires:
  MATLAB Function1/1(dotOmega) -> Integrator1/1, [dotOmega]
  [dotOmega] -> dotOmega2/1
  Integrator1/1 -> Angular Velocity Conversion/1, [Omega], Scope2/1
  Angular Velocity Conversion/1 -> Scope1/1, Omega_deg/1
  Clock/1 -> MATLAB Function1/4(t)
  [R] -> R/1
  [Omega] -> Omega/1
  u/1 -> MATLAB Function1/3(u)
  [R] -> MATLAB Function/1(R)
  [Omega] -> MATLAB Function1/2(Omega)
  Constant2/1 -> Integrator1/2
  MATLAB Function/1(dotR) -> Integrator/1
  [Omega] -> MATLAB Function/2(Omega)
  Constant1/1 -> MATLAB Function1/1(J)
  Integrator/1 -> Scope/1, [R]
  Constant3/1 -> Integrator/2

== matlab function SO3_model_AIS/MSS/Spacecraft1/MATLAB Function1 ==
  data: J input; dotOmega output; Omega input; u input; t input
function dotOmega = fcn(J, Omega, u, t)
    Omega_x = [0 -Omega(3) Omega(2);
              Omega(3) 0  -Omega(1);
              -Omega(2) Omega(1) 0];
    d=10^-3*[-1+3*sin(0.1*t+pi/2)+4*sin(0.003*t); 
    1.5-1.5*sin(0.02*t)-3*sin(0.05*t+pi/2);
    1+2*sin(0.1*t)-1.5*sin(0.04*t+pi/2)];
   dotOmega=zeros(3,1);
    dotOmega = J\(u-Omega_x*J*Omega+d);
%     dotOmega = J\(u-Omega_x*J*Omega);

== matlab function SO3_model_AIS/MSS/Spacecraft1/MATLAB Function ==
  data: R input; dotR output; Omega input
function dotR  = fcn(R, Omega)
    Omega_x = [0 -Omega(3) Omega(2);
              Omega(3) 0  -Omega(1);
              -Omega(2) Omega(1) 0];
%           [x1,y1]=eig(R);
%           
%           n=real(x1(:,3));
%           a=R*n-n;
%           theta = acos((trace(R)-1)/2);

    dotR = R*Omega_x;

== matlab function SO3_model_AIS/Controller/Controller3 ==
  settings: updateMethod=DISCRETE
  data: R1 input; R2 input; R3 input; Omega1 input; Omega2 input; Omega3 input; Rd input; Omegad input; R10 input; R20 input; R30 input; G input; u10_nod output; u20_nod output; u30_nod output; Psi output; t input; Psit output; Psic output; X input; thate_T input; norm_e_omega output; alpha input; lambda input; beta input; K input; theta_1 output; theta_12 output; theta_13 output; theta_2 output; theta_21 output; theta_23 output; theta_3 output; theta_31 output; theta_32 output; tel_I1 output; ant_I1 output; tel_I2 output; ant_I2 output; tel_I3 output; ant_I3 output; SFZ2 output; SMZ1 output; k_1 input; dot_k_1 output; k_2 input; k_3 input; dot_k_2 output; dot_k_3 output
function [u10_nod,u20_nod,u30_nod,Psi,Psit,Psic,norm_e_omega,theta_1,theta_12,...
    theta_13,theta_2,theta_21,theta_23,theta_3,theta_31,theta_32,...
    tel_I1,ant_I1,tel_I2,ant_I2,tel_I3,ant_I3,SFZ2,SMZ1,dot_k_1,dot_k_2,dot_k_3]...
    = fcn(R1,R2,R3,Omega1,Omega2,Omega3,Rd,Omegad,R10,R20,R30,G,t,X,thate_T,alpha,lambda,beta,K,k_1,k_2,k_3)
% X = n*4, 4= 1*3+1;
    %% Attitude Error Function
    Psi=zeros(3,1);
    Psit=zeros(3,1);
    Psic=zeros(3,1);
    norm_e_omega=zeros(3,1);
    
    Psit1 =0.5*trace(G*(eye(3)-Rd'*R1));
    Psit2 =0.5*trace(G*(eye(3)-Rd'*R2));
    Psit3 =0.5*trace(G*(eye(3)-Rd'*R3));
    Psit = [Psit1;Psit2;Psit3];
    
    Psic1 =0.5*trace(G*(eye(3)-R3'*R1))+0.5*trace(G*(eye(3)-R2'*R1));
    Psic2 =0.5*trace(G*(eye(3)-R1'*R2))+0.5*trace(G*(eye(3)-R3'*R2));
    Psic3 =0.5*trace(G*(eye(3)-R2'*R3))+0.5*trace(G*(eye(3)-R1'*R3));
    Psic = [Psic1;Psic2;Psic3];
    
    Psi1 = Psit1+Psic1;
    Psi2 = Psic2;
    Psi3 = Psic3;
    
    Psi = [Psi1;Psi2;Psi3];
    
    e_R12c=0.5*x_hat2x(G*R2'*R1-R1'*R2*G);
    e_R13c=0.5*x_hat2x(G*R3'*R1-R1'*R3*G);
    e_R1c = e_R12c+e_R13c;
    e_R1t =0.5*x_hat2x(G*Rd'*R1-R1'*Rd*G);
    e_R1 = e_R1c+e_R1t;
    
    e_R21c=0.5*x_hat2x(G*R1'*R2-R2'*R1*G);
    e_R23c=0.5*x_hat2x(G*R3'*R2-R2'*R3*G);
    e_R2c = e_R21c+e_R23c;
    e_R2t = 0*x_hat2x(G*Rd'*R2-R2'*Rd*G);
    e_R2 = e_R2c+e_R2t;
    
    e_R31c=0.5*x_hat2x(G*R1'*R3-R3'*R1*G);
    e_R32c=0.5*x_hat2x(G*R2'*R3-R3'*R2*G);
    e_R3c = e_R31c+e_R32c;
    e_R3t = 0*x_hat2x(G*Rd'*R3-R3'*Rd*G);
    e_R3 = e_R3c+e_R3t;
    
    e_omega_c_12=Omega1-R1'*R2*Omega2;
    e_omega_c_13=Omega1-R1'*R3*Omega3;
    e_omega_c_1=e_omega_c_12+e_omega_c_13;
    e_omega_t_1=Omega1-R1'*Rd*Omegad;
    e_omega_1 = e_omega_c_1+e_omega_t_1;
    
    e_omega_c_21=Omega2-R2'*R1*Omega1;
    e_omega_c_23=Omega2-R2'*R3*Omega3;
    e_omega_c_2=e_omega_c_21+e_omega_c_23;
    e_omega_t_2=Omega2-R2'*Rd*Omegad;
    e_omega_2 = e_omega_c_2+e_omega_t_2;
    
    e_omega_c_31=Omega3-R3'*R1*Omega1;
    e_omega_c_32=Omega3-R3'*R2*Omega2;
    e_omega_c_3=e_omega_c_31+e_omega_c_32;
    e_omega_t_3=Omega3-R3'*Rd*Omegad;
    e_omega_3 = e_omega_c_3+e_omega_t_3;
    
    norm_e_omega=[norm(e_omega_1);norm(e_omega_2);norm(e_omega_3)];
    
    %% Attitude Error Dynamics
%     dot_Psic1 = e_omega_c_12'*e_R12c+e_omega_c_13'*e_R13c;
%     dot_Psit1 = e_omega_t_1'*e_R1t;
%     dot_Psi1 = dot_Psic1+dot_Psit1;
%     
%     dot_Psic2 = e_omega_c_21'*e_R21c+e_omega_c_23'*e_R23c;
%     dot_Psit2 = e_omega_t_2'*e_R2t;
%     dot_Psi2 = dot_Psic2+dot_Psit2;
%     
%     dot_Psic3 = e_omega_c_31'*e_R31c+e_omega_c_31'*e_R32c;
%     dot_Psit3 = e_omega_t_3'*e_R3t;
%     dot_Psi3 = dot_Psic3+dot_Psit3;
    
    %% Mixed attitude constraints
%     tel = [0.750,0.433,0.500]'; %telescope
%     tel = [0,0,1]'; %telescope
%     ant = [0,1,0]'; %antenna

% tel = [0.750,0.433,0.500]'; %telescope
    tel = [0,0,1]'; %telescope
    ant = [0,1,0]'; %antenna
%     tru= [-1,0,0;0,-1,0;0,0,-1];  %three trust
tru= [-1,0,0;0,-1,0;0.750,0.433,0.500];  %three trust
    
    tel_Id = zeros(3,1);
    ant_Id = zeros(3,1);
    
    tel_I1 = zeros(3,1);
    ant_I1 = zeros(3,1);
    
    tel_I2 = zeros(3,1);
    ant_I2 = zeros(3,1);
    
    tel_I3 = zeros(3,1);
    ant_I3 = zeros(3,1);
    
    tel_Id = Rd*tel;
    ant_Id = Rd*ant;
    
    tel_I1 = R1*tel;
    ant_I1 = R1*ant;
    
    tel_I2 = R2*tel;
    ant_I2 = R2*ant;
    
    tel_I3 = R3*tel;
    ant_I3 = R3*ant;
    
    
    Phi1 = 1;
    P_Phi1 = zeros(3,1);
    Phi2 = 1;
    P_Phi2 = zeros(3,1);
    Phi3 = 1;
    P_Phi3 = zeros(3,1);
    n=(size(X,1)+1);
    
    P_DF1=0;
    P_DF2=0;
    P_DF3=0;
    theta_1=zeros(4,1);
    theta_12=zeros(3,1);
    theta_13=zeros(3,1);
    
    theta_2=zeros(4,1);
    theta_21=zeros(3,1);
    theta_23=zeros(3,1);
    
    theta_3=zeros(4,1);
    theta_31=zeros(3,1);
    theta_32=zeros(3,1);
    
for i = 1:n
    if i<n-1 % static attitude-forbidden zones
         if (cos(X(i,end))-tel'*R10'*X(i,1:3)')>0
         Phi1 = Phi1  + (-alpha * log((cos(X(i,end))-tel'*R1'*X(i,1:3)')/(1+cos(X(i,end)))));
         P_Phi1 = P_Phi1 ...
                          + (alpha*(x2x_hat(R1'*X(i,1:3)')*tel)/(tel'*R1'*X(i,1:3)'-cos(X(i,end))));
         else
         Phi1=Phi1+alpha*(tel'*R1'*X(i,1:3)'-cos(pi))^2/2;
         P_Phi1 = P_Phi1-alpha*(tel'*R1'*X(i,1:3)'-cos(pi))*(x2x_hat(R1'*X(i,1:3)')*tel);
         end
        theta_1(i)=rad2deg(acos(tel'*R1'*X(i,1:3)'));
       
        if (cos(X(i,end))-tel'*R20'*X(i,1:3)')>0
            Phi2 = Phi2  + (-alpha * log((cos(X(i,end))-tel'*R2'*X(i,1:3)')/(1+cos(X(i,end)))));
            P_Phi2 = P_Phi2 ...
                + (alpha*(x2x_hat(R2'*X(i,1:3)')*tel)/(tel'*R2'*X(i,1:3)'-cos(X(i,end))));
        else
             Phi2=Phi2+alpha*(tel'*R2'*X(i,1:3)'-cos(pi))^2/2;
             P_Phi2 = P_Phi2-alpha*(tel'*R2'*X(i,1:3)'-cos(pi))*(x2x_hat(R2'*X(i,1:3)')*tel);
        end
        
        theta_2(i)=rad2deg(acos(tel'*R2'*X(i,1:3)'));
        
        
        if (cos(X(i,end))-tel'*R30'*X(i,1:3)')>0
            Phi3 = Phi3  + (-alpha * log((cos(X(i,end))-tel'*R3'*X(i,1:3)')/(1+cos(X(i,end)))));
            P_Phi3 = P_Phi3 ...
                + (alpha*(x2x_hat(R3'*X(i,1:3)')*tel)/(tel'*R3'*X(i,1:3)'-cos(X(i,end))));
        else
            Phi3=Phi3+alpha*(tel'*R3'*X(i,1:3)'-cos(pi))^2/2;
             P_Phi3 = P_Phi3-alpha*(tel'*R3'*X(i,1:3)'-cos(pi))*(x2x_hat(R3'*X(i,1:3)')*tel);
        end
         theta_3(i)=rad2deg(acos(tel'*R3'*X(i,1:3)'));
    end
    if i==n-1 % the attitude-mandatory zones
        
        if (ant'*R10'*X(i,1:3)'-cos(X(i,end)))>0
            Phi1 = Phi1  + (-lambda * log((ant'*R1'*X(i,1:3)'-cos(X(i,end)))/(1+cos(X(i,end)))));
            P_Phi1 = P_Phi1 ...
                + (lambda*(x2x_hat(R1'*X(i,1:3)')*ant)/(ant'*R1'*X(i,1:3)'-cos(X(i,end))));
        else
            Phi1 = Phi1 + lambda*(cos(0)-ant'*R1'*X(i,1:3)')^2/2;
            P_Phi1 = P_Phi1+lambda *(cos(0)-ant'*R1'*X(i,1:3)')*(x2x_hat(R1'*X(i,1:3)')*ant);
        end    
        theta_1(i)=rad2deg(acos(ant'*R1'*X(i,1:3)'));
        
        if (ant'*R20'*X(i,1:3)'-cos(X(i,end)))>0
            Phi2 = Phi2  + (-lambda * log((ant'*R2'*X(i,1:3)'-cos(X(i,end)))/(1+cos(X(i,end)))));
            P_Phi2 = P_Phi2 ...
                + (lambda*(x2x_hat(R2'*X(i,1:3)')*ant)/(ant'*R2'*X(i,1:3)'-cos(X(i,end))));
        else
            Phi2 = Phi2 + lambda*(cos(0)-ant'*R2'*X(i,1:3)')^2/2;
            P_Phi2 = P_Phi2+lambda *(cos(0)-ant'*R2'*X(i,1:3)')*(x2x_hat(R2'*X(i,1:3)')*ant);
        end
        theta_2(i)=rad2deg(acos(ant'*R2'*X(i,1:3)'));
        
        if (ant'*R30'*X(i,1:3)'-cos(X(i,end)))>0
        Phi3 = Phi3  + (-lambda * log((ant'*R3'*X(i,1:3)'-cos(X(i,end)))/(1+cos(X(i,end)))));
        P_Phi3 = P_Phi3 ...
            + (lambda*(x2x_hat(R3'*X(i,1:3)')*ant)/(ant'*R3'*X(i,1:3)'-cos(X(i,end))));
        else
        Phi3 = Phi3 + lambda*(cos(0)-ant'*R3'*X(i,1:3)')^2/2;
        P_Phi3 = P_Phi3+lambda *(cos(0)-ant'*R3'*X(i,1:3)')*(x2x_hat(R3'*X(i,1:3)')*ant);
        end
        theta_3(i)=rad2deg(acos(ant'*R3'*X(i,1:3)'));
    end
    if i==n % relative dynamic attitude-forbidden zones
        for j=1:3 % three trust
            if (cos(thate_T)-tel'*R10'*R20*tru(j,:)')>0
                Phi1 = Phi1  + (-beta * log((cos(thate_T)-tel'*R1'*R2*tru(j,:)')/(1+cos(thate_T))));
                P_Phi1 = P_Phi1 ...
                    + (beta*(x2x_hat(R1'*R2*tru(j,:)')*tel)/(tel'*R1'*R2*tru(j,:)'-cos(thate_T)));
                P_DF1= P_DF1+ (R1'*R2*Omega2)'*(beta*(x2x_hat(R1'*R2*tru(j,:)')*tel)/(tel'*R1'*R2*tru(j,:)'-cos(thate_T)));
            else
                Phi1 = Phi1  + beta *((tel'*R1'*R2*tru(j,:)'-cos(pi))^2/2);
                P_Phi1 = P_Phi1- (beta*(tel'*R1'*R2*tru(j,:)'-cos(pi))*(x2x_hat(R1'*R2*tru(j,:)')*tel));
                P_DF1= P_DF1+ (R1'*R2*Omega2)'*(-(beta*(tel'*R1'*R2*tru(j,:)'-cos(pi))*(x2x_hat(R1'*R2*tru(j,:)')*tel)));
            end
            
            if (cos(thate_T)-tel'*R10'*R30*tru(j,:)')>0
                Phi1 = Phi1  + (-beta * log((cos(thate_T)-tel'*R1'*R3*tru(j,:)')/(1+cos(thate_T))));
                P_Phi1 = P_Phi1 ...
                    + (beta*(x2x_hat(R1'*R3*tru(j,:)')*tel)/(tel'*R1'*R3*tru(j,:)'-cos(thate_T)));
                P_DF1= P_DF1+ (R1'*R3*Omega3)'*(beta*(x2x_hat(R1'*R3*tru(j,:)')*tel)/(tel'*R1'*R3*tru(j,:)'-cos(thate_T)));
            else
                Phi1 = Phi1  + beta *((tel'*R1'*R3*tru(j,:)'-cos(pi))^2/2);
                P_Phi1 = P_Phi1- (beta*(tel'*R1'*R3*tru(j,:)'-cos(pi))*(x2x_hat(R1'*R3*tru(j,:)')*tel));
                P_DF1= P_DF1+ (R1'*R3*Omega3)'*(-(beta*(tel'*R1'*R3*tru(j,:)'-cos(pi))*(x2x_hat(R1'*R3*tru(j,:)')*tel)));
            end
            A=tel'*R1'/norm(tel'*R1');
            B=R2*tru(j,:)'/norm(R2*tru(j,:)');

            theta_12(j)=rad2deg(acos(A*B));
%             theta_13(j)=rad2deg(acos(tel'*R1'*R3*tru(j,:)'));       
%             if abs(tel'*R1'*R2*tru(j,:)')>1
%                theta_12(j)=rad2deg(acos(sign(tel'*R1'*R2*tru(j,:)'))); 
%             else
%                theta_12(j)=rad2deg(acos(tel'*R1'*R2*tru(j,:)'));
%             end
            if abs(tel'*R1'*R3*tru(j,:)')>1
               theta_13(j)=rad2deg(acos(sign(tel'*R1'*R3*tru(j,:)'))); 
            else
               theta_13(j)=rad2deg(acos(tel'*R1'*R3*tru(j,:)'));
            end        
                   
            if (cos(thate_T)-tel'*R20'*R10*tru(j,:)')>0
                Phi2 = Phi2  + (-beta * log((cos(thate_T)-tel'*R2'*R1*tru(j,:)')/(1+cos(thate_T))));
                P_Phi2 = P_Phi2 ...
                    + (beta*(x2x_hat(R2'*R1*tru(j,:)')*tel)/(tel'*R2'*R1*tru(j,:)'-cos(thate_T)));
                P_DF2= P_DF2+ (R2'*R1*Omega1)'*(beta*(x2x_hat(R2'*R1*tru(j,:)')*tel)/(tel'*R2'*R1*tru(j,:)'-cos(thate_T)));
            else
                Phi2 = Phi2  + beta *((tel'*R2'*R1*tru(j,:)'-cos(pi))^2/2);
                P_Phi2 = P_Phi2- (beta*(tel'*R2'*R1*tru(j,:)'-cos(pi))*(x2x_hat(R2'*R1*tru(j,:)')*tel));
                P_DF2= P_DF2+ (R2'*R1*Omega1)'*(-(beta*(tel'*R2'*R1*tru(j,:)'-cos(pi))*(x2x_hat(R2'*R1*tru(j,:)')*tel)));
            end

            if (cos(thate_T)-tel'*R20'*R30*tru(j,:)')>0
                Phi2 = Phi2  + (-beta * log((cos(thate_T)-tel'*R2'*R3*tru(j,:)')/(1+cos(thate_T))));
                P_Phi2 = P_Phi2 ...
                    + (beta*(x2x_hat(R2'*R3*tru(j,:)')*tel)/(tel'*R2'*R3*tru(j,:)'-cos(thate_T)));
                P_DF2= P_DF2+ (R2'*R3*Omega3)'*(beta*(x2x_hat(R2'*R3*tru(j,:)')*tel)/(tel'*R2'*R3*tru(j,:)'-cos(thate_T)));
            else
                Phi2 = Phi2  + beta *((tel'*R2'*R3*tru(j,:)'-cos(pi))^2/2);
                P_Phi2 = P_Phi2- (beta*(tel'*R2'*R3*tru(j,:)'-cos(pi))*(x2x_hat(R2'*R3*tru(j,:)')*tel));
                P_DF2= P_DF2+ (R2'*R3*Omega3)'*(-(beta*(tel'*R2'*R3*tru(j,:)'-cos(pi))*(x2x_hat(R2'*R3*tru(j,:)')*tel)));
            end

            if t>160&&j==3
                a=6;
            end
%             theta_21(j)=rad2deg(acos(tel'*R2'*R1*tru(j,:)'));
%             theta_23(j)=rad2deg(acos(tel'*R2'*R3*tru(j,:)'));
            
            if abs(tel'*R2'*R1*tru(j,:)')>1
               theta_21(j)=rad2deg(acos(sign(tel'*R2'*R1*tru(j,:)'))); 
            else
                theta_21(j)=rad2deg(acos(tel'*R2'*R1*tru(j,:)'));
            end
            if abs(tel'*R2'*R3*tru(j,:)')>1
               theta_23(j)=rad2deg(acos(sign(tel'*R3'*R2*tru(j,:)'))); 
            else
               theta_23(j)=rad2deg(acos(tel'*R2'*R3*tru(j,:)'));
            end       
                   
             if (cos(thate_T)-tel'*R30'*R10*tru(j,:)')>0
                Phi3 = Phi3  + (-beta * log((cos(thate_T)-tel'*R3'*R1*tru(j,:)')/(1+cos(thate_T))));
                P_Phi3 = P_Phi3 ...
                    + (beta*(x2x_hat(R3'*R1*tru(j,:)')*tel)/(tel'*R3'*R1*tru(j,:)'-cos(thate_T)));
                P_DF3= P_DF3+ (R3'*R1*Omega1)'*(beta*(x2x_hat(R3'*R1*tru(j,:)')*tel)/(tel'*R3'*R1*tru(j,:)'-cos(thate_T)));
            else
                Phi3 = Phi3  + beta *((tel'*R3'*R1*tru(j,:)'-cos(pi))^2/2);
                P_Phi3 = P_Phi3- (beta*(tel'*R3'*R1*tru(j,:)'-cos(pi))*(x2x_hat(R3'*R1*tru(j,:)')*tel));
                P_DF3= P_DF3+ (R3'*R1*Omega1)'*(-(beta*(tel'*R3'*R1*tru(j,:)'-cos(pi))*(x2x_hat(R3'*R1*tru(j,:)')*tel)));
             end
             
            if (cos(thate_T)-tel'*R30'*R20*tru(j,:)')>0
                Phi3 = Phi3  + (-beta * log((cos(thate_T)-tel'*R3'*R2*tru(j,:)')/(1+cos(thate_T))));
                P_Phi3 = P_Phi3 ...
                    + (beta*(x2x_hat(R3'*R2*tru(j,:)')*tel)/(tel'*R3'*R2*tru(j,:)'-cos(thate_T)));
                P_DF3= P_DF3+ (R3'*R2*Omega2)'*(beta*(x2x_hat(R3'*R2*tru(j,:)')*tel)/(tel'*R3'*R2*tru(j,:)'-cos(thate_T)));
            else
                Phi3 = Phi3  + beta *((tel'*R3'*R2*tru(j,:)'-cos(pi))^2/2);
                P_Phi3 = P_Phi3- (beta*(tel'*R3'*R2*tru(j,:)'-cos(pi))*(x2x_hat(R3'*R2*tru(j,:)')*tel));
                P_DF3= P_DF3+ (R3'*R2*Omega2)'*(-(beta*(tel'*R3'*R2*tru(j,:)'-cos(pi))*(x2x_hat(R3'*R2*tru(j,:)')*tel)));
            end
            if abs(tel'*R3'*R1*tru(j,:)')>1
               theta_31(j)=rad2deg(acos(sign(tel'*R3'*R1*tru(j,:)'))); 
            else
                theta_31(j)=rad2deg(acos(tel'*R3'*R1*tru(j,:)'));
            end
            if abs(tel'*R3'*R2*tru(j,:)')>1
               theta_32(j)=rad2deg(acos(sign(tel'*R3'*R2*tru(j,:)'))); 
            else
                theta_32(j)=rad2deg(acos(tel'*R3'*R2*tru(j,:)'));
            end
        end
    end
end

SFZ2=[theta_1(3);theta_2(3);theta_3(3)];
SMZ1=[theta_1(4);theta_2(4);theta_3(4)];

%% 传统不考虑饱和控制器
ksi=0.01; % 滑模平滑项
% if t>400
%     K(4)=0.01;
% end
dot_k_1=zeros(3,1);
dot_k_1(1)=-(K(1)*K(5)*k_1(1))/((norm(Omega1))^2+k_1(1)^2)*Psi1;
S1_1=(Omega1)/((norm(Omega1))^2+k_1(1)^2);

dot_k_1(2)=-(K(2)*K(6)*k_1(2)*(norm(Omega1)))/((norm(Omega1))+k_1(2)^2)*norm(e_omega_1);
S2_1=(Omega1)/((norm(Omega1))+k_1(2)^2);

A1=(R1'*R2*Omega2)'*e_R12c+(R1'*R3*Omega3)'*e_R13c;
M1=Psi1*P_DF1+Phi1*A1+Phi1*((R1'*Rd*Omegad)'*e_R1t);
dot_k_1(3)=(K(4)*K(7)*k_1(3))/((norm(Omega1))^2+k_1(3)^2)*M1;
S3_1=(Omega1)/((norm(Omega1))^2+k_1(3)^2);

F1=e_R1*Phi1+Psi1*P_Phi1;
u10_nod=-K(1)*Psi1*S1_1-K(2)*norm(e_omega_1)*S2_1-K(3)*(e_omega_1)-K(4)*F1+K(4)*M1*S3_1; %no disturbence


dot_k_2=zeros(3,1);
dot_k_2(1)=-(K(1)*K(5)*k_2(1))/((norm(Omega2))^2+k_2(1)^2)*Psi2;
S1_2=(Omega2)/((norm(Omega2))^2+k_2(1)^2);

dot_k_2(2)=-(K(2)*K(6)*k_2(2)*(norm(Omega2)))/((norm(Omega2))+k_2(2)^2)*norm(e_omega_2);
S2_2=(Omega2)/((norm(Omega2))+k_2(2)^2);

A2=(R2'*R1*Omega1)'*e_R21c+(R2'*R3*Omega3)'*e_R23c;
M2=Psi2*P_DF2+Phi2*A2;
dot_k_2(3)=(K(4)*K(7)*k_2(3))/((norm(Omega2))^2+k_2(3)^2)*M2;
S3_2=(Omega2)/((norm(Omega2))^2+k_2(3)^2);

F2=e_R2*Phi2+Psi2*P_Phi2;

u20_nod=-K(1)*Psi2*S1_2-K(2)*norm(e_omega_2)*S2_2-K(3)*(e_omega_2)-K(4)*F2+K(4)*M2*S3_2; %no disturbence


dot_k_3=zeros(3,1);

dot_k_3(1)=-(K(1)*K(5)*k_3(1))/((norm(Omega3))^2+k_3(1)^2)*Psi3;
S1_3=(Omega3)/((norm(Omega3))^2+k_3(1)^2);

dot_k_3(2)=-(K(2)*K(6)*k_3(2)*(norm(Omega3)))/((norm(Omega3))+k_3(2)^2)*norm(e_omega_3);
S2_3=(Omega3)/((norm(Omega3))+k_3(2)^2);

A3=(R3'*R1*Omega1)'*e_R31c+(R3'*R2*Omega2)'*e_R32c;
M3=Psi3*P_DF3+Phi3*A3;
dot_k_3(3)=(K(4)*K(7)*k_3(3))/((norm(Omega3))^2+k_3(3)^2)*M3;
S3_3=(Omega3)/((norm(Omega3))^2+k_3(3)^2);

F3=e_R3*Phi3+Psi3*P_Phi3;
u30_nod=-K(1)*Psi3*S1_3-K(2)*norm(e_omega_3)*S2_3-K(3)*(e_omega_3)-K(4)*F3+K(4)*M3*S3_3; %no disturbence
end

== matlab function SO3_model_AIS/MSS/Spacecraft2/MATLAB Function ==
  data: R input; dotR output; Omega input
function dotR  = fcn(R, Omega)
    Omega_x = [0 -Omega(3) Omega(2);
              Omega(3) 0  -Omega(1);
              -Omega(2) Omega(1) 0];
%           [x1,y1]=eig(R);
%           
%           n=real(x1(:,3));
%           a=R*n-n;
%           theta = acos((trace(R)-1)/2);

    dotR = R*Omega_x;

== matlab function SO3_model_AIS/MSS/Spacecraft2/MATLAB Function1 ==
  data: J input; dotOmega output; Omega input; u input; t input
function dotOmega = fcn(J, Omega, u, t)
    Omega_x = [0 -Omega(3) Omega(2);
              Omega(3) 0  -Omega(1);
              -Omega(2) Omega(1) 0];
    d=10^-3*[-1+3*sin(0.1*t+pi/2)+4*sin(0.003*t);
    1.5-1.5*sin(0.02*t)-3*sin(0.05*t+pi/2);
    1+2*sin(0.1*t)-1.5*sin(0.04*t+pi/2)];
    dotOmega=zeros(3,1);
    dotOmega = J\(u-Omega_x*J*Omega+d);
%     dotOmega = J\(u-Omega_x*J*Omega);

== matlab function SO3_model_AIS/MSS/Spacecraft3/MATLAB Function ==
  data: R input; dotR output; Omega input
function dotR  = fcn(R, Omega)
    Omega_x = [0 -Omega(3) Omega(2);
              Omega(3) 0  -Omega(1);
              -Omega(2) Omega(1) 0];
%           [x1,y1]=eig(R);
%           
%           n=real(x1(:,3));
%           a=R*n-n;
%           theta = acos((trace(R)-1)/2);

    dotR = R*Omega_x;

== matlab function SO3_model_AIS/MSS/Spacecraft3/MATLAB Function1 ==
  data: J input; dotOmega output; Omega input; u input; t input
function dotOmega = fcn(J, Omega, u, t)
    Omega_x = [0 -Omega(3) Omega(2);
              Omega(3) 0  -Omega(1);
              -Omega(2) Omega(1) 0];
    d=10^-3*[-1+3*sin(0.1*t+pi/2)+4*sin(0.003*t);
    1.5-1.5*sin(0.02*t)-3*sin(0.05*t+pi/2);
    1+2*sin(0.1*t)-1.5*sin(0.04*t+pi/2)];
    dotOmega=zeros(3,1);
    dotOmega = J\(u-Omega_x*J*Omega+d);
%     dotOmega = J\(u-Omega_x*J*Omega);

== matlab function SO3_model_AIS/Controller/Subsystem/MATLAB Function ==
  data: u0_d1 output; u0_d2 output; u0_d3 output; Omega1 input; dot_hat_dmax1 output; Omega2 input; Omega3 input; dot_hat_dmax2 output; dot_hat_dmax3 output; hat_dmax1 input; hat_dmax2 input; hat_dmax3 input; k_d input; dot_k_d output
function [u0_d1,u0_d2,u0_d3,dot_hat_dmax1,dot_hat_dmax2,dot_hat_dmax3,dot_k_d] = fcn(Omega1,Omega2,Omega3,hat_dmax1,hat_dmax2,hat_dmax3,k_d)
    u0_d1=zeros(3,1);
    u0_d2=zeros(3,1);
    u0_d3=zeros(3,1);
    dot_hat_dmax1=0;
    dot_hat_dmax2=0;
    dot_hat_dmax3=0;

   eta3 =0.1;
   ksi3 =0.000025;
   delta3=0.00008;
   
   if hat_dmax1^2<ksi3
       dot_hat_dmax1 = eta3*norm(Omega1);
   end
   if hat_dmax1^2>=ksi3
        dot_hat_dmax1 = eta3*(norm(Omega1)-(hat_dmax1^2-ksi3)*norm(Omega1)*hat_dmax1/(delta3*hat_dmax1^2)*hat_dmax1);
   end
   
   if hat_dmax2^2<ksi3
        dot_hat_dmax2 = eta3*norm(Omega2);
   end
   if hat_dmax2^2>=ksi3
        dot_hat_dmax2 = eta3*(norm(Omega2)-(hat_dmax2^2-ksi3)*norm(Omega2)*hat_dmax2/(delta3*hat_dmax2^2)*hat_dmax2);
   end
   
   if hat_dmax3^2<ksi3
        dot_hat_dmax3 = eta3*norm(Omega3);
   end
   if hat_dmax3^2>=ksi3
        dot_hat_dmax3 = eta3*(norm(Omega3)-(hat_dmax3^2-ksi3)*norm(Omega3)*hat_dmax3/(delta3*hat_dmax3^2)*hat_dmax3);
   end
   k_8=3;
   dot_k_d=zeros(3,1);
   
   dot_k_d(1)=-(k_8*k_d(1)*(norm(Omega1)))/((norm(Omega1))+k_d(1)^2)*hat_dmax1;
   dot_k_d(2)=-(k_8*k_d(2)*(norm(Omega2)))/((norm(Omega2))+k_d(2)^2)*hat_dmax2;
   dot_k_d(3)=-(k_8*k_d(3)*(norm(Omega3)))/((norm(Omega3))+k_d(3)^2)*hat_dmax3;

  
   u0_d1 = hat_dmax1*Omega1/(norm(Omega1)+k_d(1)^2);
   u0_d2 = hat_dmax2*Omega2/(norm(Omega2)+k_d(2)^2);
   u0_d3 = hat_dmax3*Omega3/(norm(Omega3)+k_d(3)^2);

== matlab function SO3_model_AIS/Virtual leader/Spacecraft4/MATLAB Function ==
  data: R input; dotR output; Omega input
function dotR  = fcn(R, Omega)
    Omega_x = [0 -Omega(3) Omega(2);
              Omega(3) 0  -Omega(1);
              -Omega(2) Omega(1) 0];
%           [x1,y1]=eig(R);
%           
%           n=real(x1(:,3));
%           a=R*n-n;
%           theta = acos((trace(R)-1)/2);

    dotR = R*Omega_x;

== matlab function SO3_model_AIS/Virtual leader/Spacecraft4/MATLAB Function1 ==
  data: J input; dotOmega output; Omega input; u input; t input
function dotOmega = fcn(J, Omega, u, t)
    Omega_x = [0 -Omega(3) Omega(2);
              Omega(3) 0  -Omega(1);
              -Omega(2) Omega(1) 0];
    d=10^-3*[-1+3*sin(0.1*t+pi/2)+4*sin(0.003*t);
    1.5-1.5*sin(0.02*t)-3*sin(0.05*t+pi/2);
    1+2*sin(0.1*t)-1.5*sin(0.04*t+pi/2)];

%     dotOmega = J\(u-Omega_x*J*Omega+d);
    dotOmega = J\(u-Omega_x*J*Omega);
